simulink model "uavsimblockset_test_landinggear"  (Simulink 8.0)
settings: Solver=ode23  StartTime=0.0  StopTime=inf  FixedStep=1/100  RelTol=1e-3
libraries: uavsimBlockset_landinggear_onwheel x1
settings Model: Creator=Jan  LastModifiedBy=j.bolting
settings SolverCC: ZeroCrossAlgorithm=Adaptive

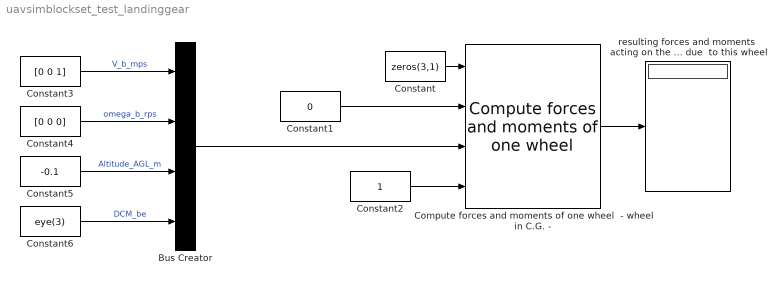
== system uavsimblockset_test_landinggear ==
  Bus Creator : BusCreator  OutDataTypeStr=Bus: LandinggearInput  NonVirtualBus=on
  Compute forces and moments of one wheel  - wheel in C.G. - : uavsimBlockset_landinggear_onwheel/Compute forces and moments of one wheel
  Constant : Constant  Value=zeros(3,1)
  Constant1 : Constant  Value=0
  Constant2 : Constant
  Constant3 : Constant  Value=[0 0 1]
  Constant4 : Constant  Value=[0 0 0]
  Constant5 : Constant  Value=-0.1
  Constant6 : Constant  Value=eye(3)
  resulting forces and moments  acting on the A\C due  to this wheel : Display
  wires:
  Compute forces and moments of one wheel  - wheel in C.G. -/1 -> resulting forces and moments  acting on the A\C due  to this wheel/1
  Constant/1 -> Compute forces and moments of one wheel  - wheel in C.G. -/1
  Constant1/1 -> Compute forces and moments of one wheel  - wheel in C.G. -/2
  Constant2/1 -> Compute forces and moments of one wheel  - wheel in C.G. -/4
  Bus Creator/1 -> Compute forces and moments of one wheel  - wheel in C.G. -/3
  Constant3/1 -> Bus Creator/1  "V_b_mps"
  Constant4/1 -> Bus Creator/2  "omega_b_rps"
  Constant5/1 -> Bus Creator/3  "Altitude_AGL_m"
  Constant6/1 -> Bus Creator/4  "DCM_be"
